simulink model "lab5_simulink"  (R2015b)
settings: Solver=ode45  StartTime=0.0  StopTime=1000  RelTol=1e-3
values from neighbouring files (symbols this model uses):
  c = [theta(4),theta(3)]    [lab2.m]    (also in lab5.m)
  g = [0,1;theta(2),theta(1)]    [lab2.m]    (also in lab5.m)
  h = [0;1]    [lab2.m]    (also in lab5.m)
  Ki = 0.025    [lab5.m]
  Kp = 0.65    [lab5.m]
libraries: simulink x2
settings Model: Creator=Charles  LastModifiedBy=My Project
settings DataIOCC: SaveFormat=Array  SignalLoggingSaveFormat=ModelDataLogs
settings OptimizationCC: ExpressionDepthLimit=2147483647
settings DebuggingCC: UnderspecifiedInitializationDetection=Classic  MergeDetectMultiDrivingBlocksExec=none  SolverPrmCheckMsg=warning  FcnCallInpInsideContextMsg=EnableAllAsWarning  AllowSymbolicDim=on  StateNameClashWarn=warning
settings HardwareCC: ProdBitPerPointer=32  ProdLargestAtomicFloat=None  ProdIntDivRoundTo=Undefined  ProdEndianess=Unspecified  ProdWordSize=32  ProdHWDeviceType=32-bit Generic
settings GRTTargetCC: GeneratePreprocessorConditionals=Disable all  CombineOutputUpdateFcns=off  GRTInterface=on
settings ConfigComp: CovModelRefEnable=Off

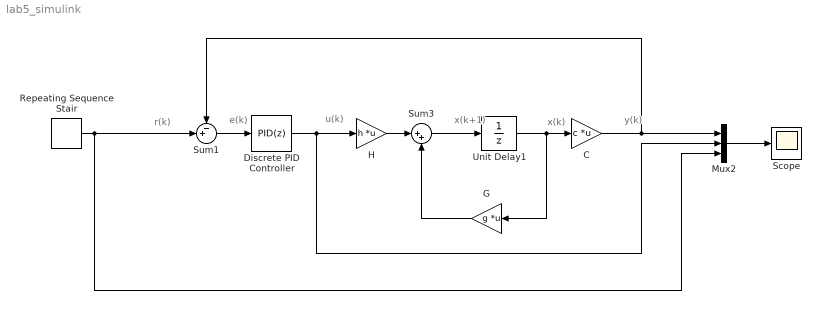
== system lab5_simulink ==
  note: r(k)
  note: e(k)
  note: u(k)
  note: y(k)
  note: x(k)
  note: x(k+1)
  C : Gain  Gain=c  Multiplication=Matrix(K*u)
  Discrete PID Controller : simulink/Continuous/PID Controller  Controller=PID  TimeDomain=Discrete-time  SampleTime=0.75  IntegratorMethod=Forward Euler  FilterMethod=Forward Euler  Form=Parallel  UseFilter=on  ControllerParametersSource=internal  P=Kp  I=Ki  D=0  N=100  InitialConditionSource=internal  InitialConditionForIntegrator=0  InitialConditionForFilter=0  ExternalReset=none  LimitOutput=off  UpperSaturationLimit=inf  LowerSaturationLimit=-inf  LinearizeAsGain=off  AntiWindupMode=none  Kb=1  TrackingMode=off  Kt=1  PParamMin=[]  PParamMax=[]  IParamMin=[]  IParamMax=[]  DParamMin=[]  DParamMax=[]  NParamMin=[]  NParamMax=[]  KbParamMin=[]  KbParamMax=[]  KtParamMin=[]  KtParamMax=[]  POutMin=[]  POutMax=[]  IOutMin=[]  IOutMax=[]  DOutMin=[]  DOutMax=[]  NOutMin=[]  NOutMax=[]  KbOutMin=[]  KbOutMax=[]  KtOutMin=[]  KtOutMax=[]  IntegratorOutMin=[]  IntegratorOutMax=[]  FilterOutMin=[]  FilterOutMax=[]  SumOutMin=[]  SumOutMax=[]  SumI1OutMin=[]  SumI1OutMax=[]  SumI2OutMin=[]  SumI2OutMax=[]  SumI3OutMin=[]  SumI3OutMax=[]  SumDOutMin=[]  SumDOutMax=[]  SaturationOutMin=[]  SaturationOutMax=[]  IntegratorContinuousStateAttributes=''  IntegratorStateMustResolveToSignalObject=off  IntegratorRTWStateStorageClass=Auto  FilterContinuousStateAttributes=''  FilterStateMustResolveToSignalObject=off  FilterRTWStateStorageClass=Auto  DifferentiatorICPrevScaledInput=0  DifferentiatorOutMin=[]  DifferentiatorOutMax=[]
  G : Gain  Gain=g  Multiplication=Matrix(K*u)
  H : Gain  Gain=h  Multiplication=Matrix(K*u)
  Mux2 : Mux  Inputs=3
  Repeating Sequence Stair : simulink/Sources/Repeating Sequence Stair  OutValues=[ 0 0.7 0.2 -0.5 0]  tsamp=140*0.75  OutMin=[]  OutMax=[]  OutDataTypeStr=double  OutputDataTypeScalingMode=double  OutDataType=fixdt(0,8)  ConRadixGroup=Best Precision: Vector-wise  OutScaling=2^-12
  Scope : Scope
  Sum1 : Sum  Inputs=-+|
  Sum3 : Sum  Inputs=|++
  Unit Delay1 : UnitDelay  SampleTime=0.75
  wires:
  H/1 -> Sum3/1
  Sum3/1 -> Unit Delay1/1
  Unit Delay1/1 -> C/1, G/1
  G/1 -> Sum3/2
  Sum1/1 -> Discrete PID Controller/1
  Mux2/1 -> Scope/1
  C/1 -> Sum1/1, Mux2/1
  Discrete PID Controller/1 -> H/1, Mux2/2
  Repeating Sequence Stair/1 -> Sum1/2, Mux2/3
